simulink model "Feedback_Linearization_LAB"  (R2022b)
settings: Solver=FixedStepDiscrete  StartTime=0.0  StopTime=60  FixedStep=0.01  RelTol=1e-3  EnableMultiTasking=on
undefined symbols (not defined in the file or in its folder): DiscIntNeverNeededParam, drv, gbox, mot, sens, Tc, Ts, wheel
libraries: BalRobTbx_baselib x9
settings Model: ExtModeTrigDuration=2  Creator=Alessandro  LastModifiedBy=david
settings SolverCC: AlgebraicLoopSolver=TrustRegion
settings OptimizationCC: EnhancedBackFolding=on  PassReuseOutputArgsAs=Individual arguments  ZeroExternalMemoryAtStartup=off  ZeroInternalMemoryAtStartup=off  MaxStackSize=64  OptimizeBlockOrder=speed  DifferentSizesBufferReuse=on  OptimizationCustomize=off  EfficientTunableParamExpr=on
settings DebuggingCC: ParameterTunabilityLossMsg=error
settings HardwareCC: ProdBitPerInt=16  ProdBitPerPointer=16  ProdBitPerSizeT=16  ProdBitPerPtrDiffT=16  ProdLargestAtomicFloat=None  ProdWordSize=8  ProdHWDeviceType=Atmel->AVR
settings ModelReferenceCC: EnableRefExpFcnMdlSchedulingChecks=on
settings SFSimCC: MATLABDynamicMemAlloc=off
settings RTWCC: Description=Embedded Coder  SystemTargetFile=ert.tlc  HardwareBoard=Arduino Mega 2560  TLCOptions=-aInlineSetEventsForThisBaseRateFcn=TLC_FALSE -aSuppressMultiTaskScheduler=TLC_FALSE -aRateBasedStepFcn=1  TemplateMakefile=ert_default_tmf  Toolchain=Arduino AVR  BuildConfiguration=Faster Runs  DLArmComputeVersion=19.05
settings CodeAppCC: ForceParamTrailComments=on  IgnoreCustomStorageClasses=off  OperatorAnnotations=on  SimulinkDataObjDesc=on  SFDataObjDesc=on  InsertBlockDesc=on
settings ERTTargetCC: SupportContinuousTime=on  SupportVariableSizeSignals=on  ExtModeTransport=3  ExtModeStaticAlloc=on  ExtModeAutomaticAllocSize=off  ExtModeStaticAllocSize=2048  ExtModeMexFile=ext_xcp  ExtModeIntrfLevel=Level2 - Open

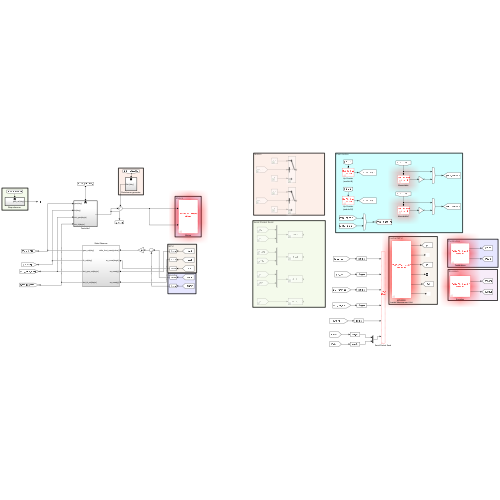
[thumbnail: Simulink's stored preview of the top-level diagram]
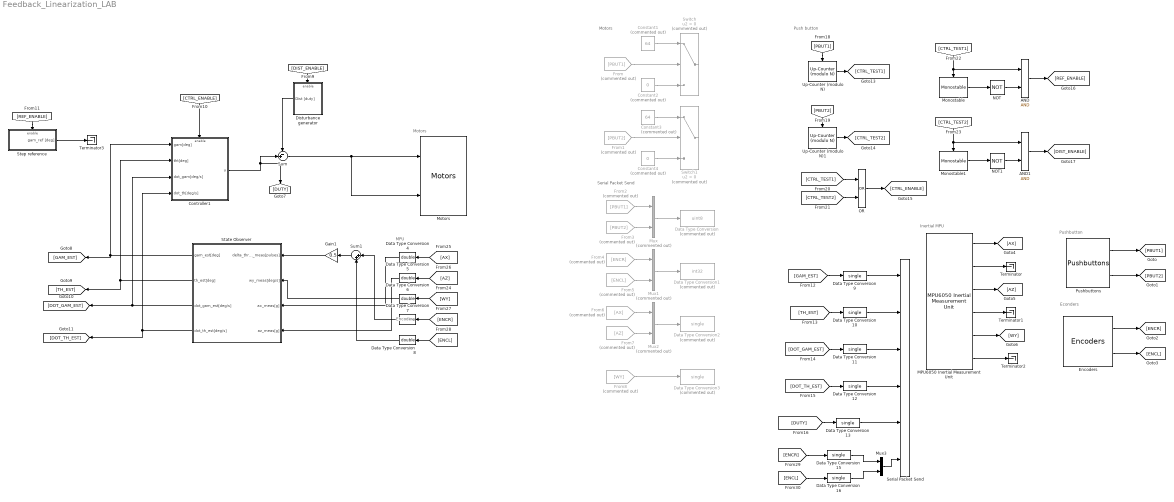
== system Feedback_Linearization_LAB ==
  note: Encoder
  note: MPU
  note: Push button
  note: Motors
  note: Serial Packet Send
  note: Econders
  note: Pushbutton
  note: Motors
  note: Inertial MPU
  AND : Logic  IconShape=distinctive  AllPortsSameDT=off  OutDataTypeStr=boolean
  AND1 : Logic  IconShape=distinctive  AllPortsSameDT=off  OutDataTypeStr=boolean
  Constant1 : Constant  Commented=on  Value=64
  Constant2 : Constant  Commented=on  Value=0
  Constant3 : Constant  Commented=on  Value=64
  Constant4 : Constant  Commented=on  Value=0
  Controller1 : Subsystem
  Data Type Conversion : DataTypeConversion  Commented=on  OutDataTypeStr=uint8  SaturateOnIntegerOverflow=off  RndMeth=Floor
  Data Type Conversion1 : DataTypeConversion  Commented=on  OutDataTypeStr=int32  SaturateOnIntegerOverflow=off  RndMeth=Floor
  Data Type Conversion{9..13,15..16} (7 alike) : DataTypeConversion  OutDataTypeStr=single  SaturateOnIntegerOverflow=off  RndMeth=Floor
  Data Type Conversion2 : DataTypeConversion  Commented=on  OutDataTypeStr=single  SaturateOnIntegerOverflow=off  RndMeth=Floor
  Data Type Conversion3 : DataTypeConversion  Commented=on  OutDataTypeStr=single  SaturateOnIntegerOverflow=off  RndMeth=Floor
  Data Type Conversion{4..8} (5 alike) : DataTypeConversion  OutDataTypeStr=double  SaturateOnIntegerOverflow=off  RndMeth=Floor
  Disturbance generator : Subsystem
  Encoders : BalRobTbx_baselib/Inputs/Encoders
  From : From  Commented=on  GotoTag=PBUT1
  From1 : From  Commented=on  GotoTag=PBUT2
  From2 : From  Commented=on  GotoTag=PBUT1
  From3 : From  Commented=on  GotoTag=PBUT2
  From4 : From  Commented=on  GotoTag=ENCR
  From5 : From  Commented=on  GotoTag=ENCL
  From6 : From  Commented=on  GotoTag=AX
  From7 : From  Commented=on  GotoTag=AZ
  From8 : From  Commented=on  GotoTag=WY
  Gain1 : Gain  Gain=0.5
  MPU6050 Inertial Measurement Unit : BalRobTbx_baselib/Inputs/MPU6050 Inertial Measurement Unit
  Monostable : BalRobTbx_baselib/Utilities/Monostable  Tp=1
  Monostable1 : BalRobTbx_baselib/Utilities/Monostable  Tp=1
  Motors : BalRobTbx_baselib/Outputs/Motors
  Mux : Mux  Commented=on  Inputs=2
  Mux1 : Mux  Commented=on  Inputs=2
  Mux2 : Mux  Commented=on  Inputs=2
  Mux3 : Mux  Inputs=2
  NOT : Logic  Operator=NOT  IconShape=distinctive  AllPortsSameDT=off  OutDataTypeStr=boolean
  NOT1 : Logic  Operator=NOT  IconShape=distinctive  AllPortsSameDT=off  OutDataTypeStr=boolean
  OR : Logic  Operator=OR  IconShape=distinctive  AllPortsSameDT=off  OutDataTypeStr=boolean
  Pushbuttons : BalRobTbx_baselib/Inputs/Pushbuttons
  Serial Packet Send : BalRobTbx_baselib/Communication/Serial Packet Send  serialLinkOpt=Bluetooth  baudRateOpt=38400  waitHostTxCmd=on  txStartCmd=65  txStopCmd=66  packetSpec={'single','single','single','single','single','2*single'}  cobsEncoded=on  nullTerminated=on  showEnablePort=off
  State Observer : Subsystem
  "Step reference " : Subsystem
  Sum : Sum  Inputs=-+|
  Sum1 : Sum  Inputs=|++
  Switch : Switch  Commented=on  Criteria=u2 > Threshold  SaturateOnIntegerOverflow=off  InputSameDT=off
  Switch1 : Switch  Commented=on  Criteria=u2 > Threshold  SaturateOnIntegerOverflow=off  InputSameDT=off
  Terminator{,1..3} (4 alike) : Terminator
  Up-Counter (modulo N) : BalRobTbx_baselib/Utilities/Up-Counter (modulo N)  N=10  C0=0
  Up-Counter (modulo N)1 : BalRobTbx_baselib/Utilities/Up-Counter (modulo N)  N=10  C0=0
  wires:
  Controller1/1(u) -> Sum/2, [DUTY]
  State Observer/1(gam_est[deg]) -> Controller1/1(gam[deg]), [GAM_EST]
  State Observer/2(th_est[deg]) -> Controller1/2(tht[deg]), [TH_EST]
  State Observer/4(dot_th_est[deg/s]) -> Controller1/4(dot_th[deg/s]), [DOT_TH_EST]
  State Observer/3(dot_gam_est[deg/s]) -> Controller1/3(dot_gam[deg/s]), [DOT_GAM_EST]
  From2/1 -> Mux/1
  From8/1 -> Data Type Conversion3/1
  Constant1/1 -> Switch/1
  From/1 -> Switch/2
  Constant3/1 -> Switch1/1
  Mux/1 -> Data Type Conversion/1
  From6/1 -> Mux2/1
  From5/1 -> Mux1/2
  From3/1 -> Mux/2
  From4/1 -> Mux1/1
  Mux1/1 -> Data Type Conversion1/1
  Constant4/1 -> Switch1/3
  From1/1 -> Switch1/2
  Constant2/1 -> Switch/3
  Mux2/1 -> Data Type Conversion2/1
  From7/1 -> Mux2/2
  Disturbance generator/1(Dist [duty]) -> Sum/1
  [DIST_ENABLE] -> Disturbance generator/Enable
  [REF_ENABLE] -> "Step reference "/Enable
  [CTRL_TEST1] -> OR/1
  [CTRL_TEST2] -> OR/2
  OR/1 -> [CTRL_ENABLE]
  NOT/1 -> AND/2
  [CTRL_TEST1] -> Monostable/Enable, AND/1
  AND/1 -> [REF_ENABLE]
  AND1/1 -> [DIST_ENABLE]
  NOT1/1 -> AND1/2
  [CTRL_TEST2] -> Monostable1/Enable, AND1/1
  [WY] -> Data Type Conversion6/1
  [AX] -> Data Type Conversion4/1
  [AZ] -> Data Type Conversion5/1
  [ENCR] -> Data Type Conversion7/1
  [ENCL] -> Data Type Conversion8/1
  [TH_EST] -> Data Type Conversion10/1
  [GAM_EST] -> Data Type Conversion9/1
  [DOT_GAM_EST] -> Data Type Conversion11/1
  [DOT_TH_EST] -> Data Type Conversion12/1
  [DUTY] -> Data Type Conversion13/1
  Up-Counter (modulo N)/1 -> [CTRL_TEST1]
  [PBUT1] -> Up-Counter (modulo N)/Trigger
  Up-Counter (modulo N)1/1 -> [CTRL_TEST2]
  [PBUT2] -> Up-Counter (modulo N)1/Trigger
  Sum/1 -> Motors/2, Motors/1
  MPU6050 Inertial Measurement Unit/2 -> Terminator/1
  MPU6050 Inertial Measurement Unit/3 -> [AZ]
  MPU6050 Inertial Measurement Unit/4 -> Terminator1/1
  MPU6050 Inertial Measurement Unit/5 -> [WY]
  MPU6050 Inertial Measurement Unit/6 -> Terminator2/1
  MPU6050 Inertial Measurement Unit/1 -> [AX]
  Pushbuttons/2 -> [PBUT2]
  Pushbuttons/1 -> [PBUT1]
  Encoders/1 -> [ENCR]
  Encoders/2 -> [ENCL]
  Monostable/1 -> NOT/1
  Monostable1/1 -> NOT1/1
  [ENCR] -> Data Type Conversion15/1
  Data Type Conversion15/1 -> Mux3/1
  Data Type Conversion16/1 -> Mux3/2
  [ENCL] -> Data Type Conversion16/1
  Data Type Conversion13/1 -> Serial Packet Send/5
  Mux3/1 -> Serial Packet Send/6
  Data Type Conversion9/1 -> Serial Packet Send/1
  Data Type Conversion10/1 -> Serial Packet Send/2
  Data Type Conversion11/1 -> Serial Packet Send/3
  Data Type Conversion12/1 -> Serial Packet Send/4
  Gain1/1 -> State Observer/1(delta_throt_meas[pulses])
  Data Type Conversion4/1 -> State Observer/3(ax_meas[g])
  Data Type Conversion5/1 -> State Observer/4(az_meas[g])
  Data Type Conversion6/1 -> State Observer/2(wy_meas[deg/s])
  Data Type Conversion7/1 -> Sum1/1
  Data Type Conversion8/1 -> Sum1/2
  Sum1/1 -> Gain1/1
  [CTRL_ENABLE] -> Controller1/Enable
  "Step reference "/1(gam_ref [deg]) -> Terminator3/1

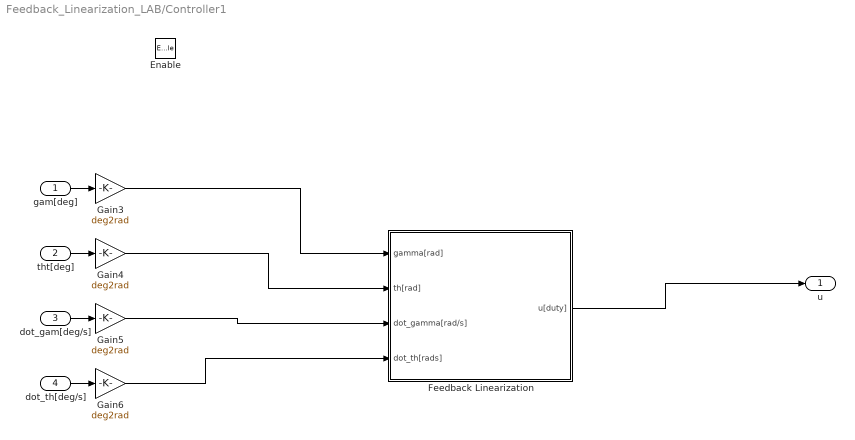
== system Feedback_Linearization_LAB/Controller1 ==
  gam[deg] : Inport
  tht[deg] : Inport  Port=2
  dot_gam[deg/s] : Inport  Port=3
  dot_th[deg/s] : Inport  Port=4
  Enable : EnablePort
  Feedback Linearization : Subsystem
  Gain{3..6} (4 alike) : Gain  Gain=deg2rad
  u : Outport  VectorParamsAs1DForOutWhenUnconnected=off
  wires:
  gam[deg]/1 -> Gain3/1
  dot_th[deg/s]/1 -> Gain6/1
  dot_gam[deg/s]/1 -> Gain5/1
  tht[deg]/1 -> Gain4/1
  Gain3/1 -> Feedback Linearization/1(gamma[rad])
  Gain4/1 -> Feedback Linearization/2(th[rad])
  Gain5/1 -> Feedback Linearization/3(dot_gamma[rad/s])
  Gain6/1 -> Feedback Linearization/4(dot_th[rads])
  Feedback Linearization/1(u[duty]) -> u/1

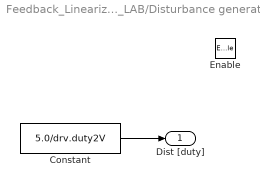
== system Feedback_Linearization_LAB/Disturbance generator ==
  Enable : EnablePort
  Constant : Constant  Value=5.0/drv.duty2V
  Dist [duty] : Outport  InitialOutput=0
  wires:
  Constant/1 -> Dist [duty]/1

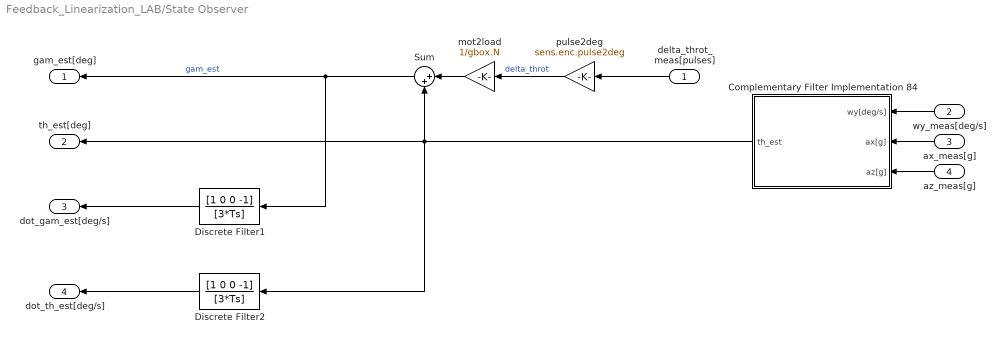
== system Feedback_Linearization_LAB/State Observer ==
  delta_throt_meas[pulses] : Inport
  wy_meas[deg/s] : Inport  Port=2
  ax_meas[g] : Inport  Port=3
  az_meas[g] : Inport  Port=4
  Complementary Filter Implementation 84 : Subsystem
  Discrete Filter1 : DiscreteFilter  Numerator=[1 0 0 -1]  Denominator=[3*Ts]  SampleTime=Ts
  Discrete Filter2 : DiscreteFilter  Numerator=[1 0 0 -1]  Denominator=[3*Ts]  SampleTime=Ts
  Sum : Sum  Inputs=|++
  mot2load : Gain  Gain=1/gbox.N
  pulse2deg : Gain  Gain=sens.enc.pulse2deg
  gam_est[deg] : Outport  VectorParamsAs1DForOutWhenUnconnected=off
  th_est[deg] : Outport  Port=2  VectorParamsAs1DForOutWhenUnconnected=off
  dot_gam_est[deg/s] : Outport  Port=3  VectorParamsAs1DForOutWhenUnconnected=off
  dot_th_est[deg/s] : Outport  Port=4  VectorParamsAs1DForOutWhenUnconnected=off
  wires:
  Sum/1 -> Discrete Filter1/1, gam_est[deg]/1  "gam_est"
  Discrete Filter2/1 -> dot_th_est[deg/s]/1
  mot2load/1 -> Sum/1
  delta_throt_meas[pulses]/1 -> pulse2deg/1
  Complementary Filter Implementation 84/1(th_est) -> Discrete Filter2/1, th_est[deg]/1, Sum/2
  pulse2deg/1 -> mot2load/1  "delta_throt"
  Discrete Filter1/1 -> dot_gam_est[deg/s]/1
  az_meas[g]/1 -> Complementary Filter Implementation 84/3(az[g])
  ax_meas[g]/1 -> Complementary Filter Implementation 84/2(ax[g])
  wy_meas[deg/s]/1 -> Complementary Filter Implementation 84/1(wy[deg/s])

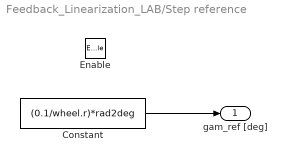
== system Feedback_Linearization_LAB/Step reference  ==
  Enable : EnablePort
  Constant : Constant  Value=(0.1/wheel.r)*rad2deg
  gam_ref [deg] : Outport
  wires:
  Constant/1 -> gam_ref [deg]/1

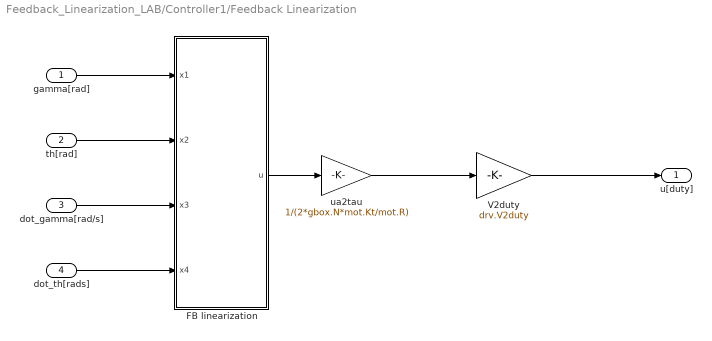
== system Feedback_Linearization_LAB/Controller1/Feedback Linearization ==
  gamma[rad] : Inport
  th[rad] : Inport  Port=2
  dot_gamma[rad/s] : Inport  Port=3
  dot_th[rads] : Inport  Port=4
  FB linearization : MATLAB Function  TreatAsAtomicUnit=on
  V2duty : Gain  Gain=drv.V2duty
  ua2tau : Gain  Gain=1/(2*gbox.N*mot.Kt/mot.R)
  u[duty] : Outport
  wires:
  FB linearization/1(u) -> ua2tau/1
  dot_th[rads]/1 -> FB linearization/4(x4)
  th[rad]/1 -> FB linearization/2(x2)
  gamma[rad]/1 -> FB linearization/1(x1)
  dot_gamma[rad/s]/1 -> FB linearization/3(x3)
  ua2tau/1 -> V2duty/1
  V2duty/1 -> u[duty]/1

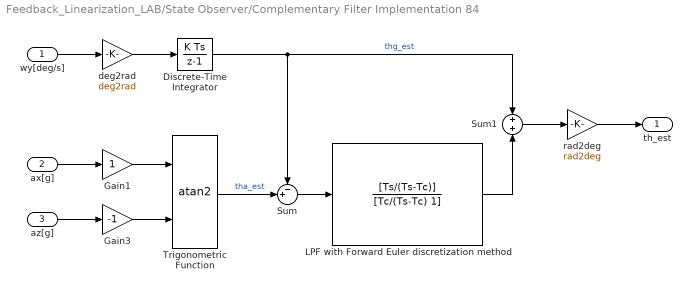
== system Feedback_Linearization_LAB/State Observer/Complementary Filter Implementation 84 ==
  wy[deg/s] : Inport
  ax[g] : Inport  Port=2
  az[g] : Inport  Port=3
  Discrete-Time Integrator : DiscreteIntegrator  SampleTime=Ts  ICPrevOutput=DiscIntNeverNeededParam  ICPrevScaledInput=DiscIntNeverNeededParam
  Gain1 : Gain
  Gain3 : Gain  Gain=-1
  LPF with Forward Euler discretization method : DiscreteTransferFcn  Numerator=[Ts/(Ts-Tc)]  Denominator=[Tc/(Ts-Tc) 1]  SampleTime=Ts
  Sum : Sum  Inputs=-+|
  Sum1 : Sum  Inputs=+|+
  Trigonometric Function : Trigonometry  Operator=atan2
  deg2rad : Gain  Gain=deg2rad
  rad2deg : Gain  Gain=rad2deg
  th_est : Outport  VectorParamsAs1DForOutWhenUnconnected=off
  wires:
  Gain3/1 -> Trigonometric Function/2
  Trigonometric Function/1 -> Sum/2  "tha_est"
  az[g]/1 -> Gain3/1
  Gain1/1 -> Trigonometric Function/1
  Discrete-Time Integrator/1 -> Sum1/1, Sum/1  "thg_est"
  deg2rad/1 -> Discrete-Time Integrator/1
  Sum1/1 -> rad2deg/1
  wy[deg/s]/1 -> deg2rad/1
  ax[g]/1 -> Gain1/1
  LPF with Forward Euler discretization method/1 -> Sum1/2
  Sum/1 -> LPF with Forward Euler discretization method/1
  rad2deg/1 -> th_est/1

== matlab function Feedback_Linearization_LAB/Controller1/Feedback Linearization/FB linearization ==
  data: x1 input; x2 input; u output; x3 input; x4 input; num1 parameter
function u   = fcn(x1, x2, x3 ,x4, num1)

f=[x3;
    x4;
    -(num1.g2*num1.m12*sin(x2) - num1.f11*num1.m22*x3 + num1.f21*num1.m12*x3 + num1.f22*num1.m12*x4 - num1.f21*num1.m22*x4 + num1.f21*num1.k*x3*cos(x2) + num1.f22*num1.k*x4*cos(x2) - num1.c12*num1.m22*x4^2*sin(x2) + num1.g2*num1.k*cos(x2)*sin(x2))/(num1.k^2*cos(x2)^2 + 2*num1.k*num1.m12*cos(x2) + num1.m12^2 - num1.m11*num1.m22);
    -(num1.f11*num1.m12*x3 - num1.g2*num1.m11*sin(x2) - num1.f21*num1.m11*x3 + num1.f21*num1.m12*x4 - num1.f22*num1.m11*x4 + num1.f11*num1.k*x3*cos(x2) + num1.f21*num1.k*x4*cos(x2) + num1.c12*num1.m12*x4^2*sin(x2) + num1.c12*num1.k*x4^2*cos(x2)*sin(x2))/(num1.k^2*cos(x2)^2 + 2*num1.k*num1.m12*cos(x2) + num1.m12^2 - num1.m11*num1.m22)];
g=[0; 0;
    -(num1.m12 + num1.m22 + num1.k*cos(x2))/(num1.k^2*cos(x2)^2 + 2*num1.k*num1.m12*cos(x2) + num1.m12^2 - num1.m11*num1.m22);
    (num1.m11 + num1.m12 + num1.k*cos(x2))/(num1.k^2*cos(x2)^2 + 2*num1.k*num1.m12*cos(x2) + num1.m12^2 - num1.m11*num1.m22)];

%K= [72 17];%poli sim2
K=[100.25, 20];% poli sim1 sim3
x1_d=0;
c= [10 5 15];
v =-K(1)*(x2)-K(2)*x4;
u=(-f(4)+v)/g(4)-((-c(1)*(x1-x1_d)-c(3)*x3-c(2)*f(3))*g(4)-c(2)*g(3)*(v-f(4)))/(c(2)*g(3)*g(4));
%u=(-f(4)+v)/g(4);
end
